simulink model "Traffic_Light"  (R2022b)
settings: Solver=VariableStepAuto  StartTime=0.0  StopTime=50  RelTol=1e-3
settings Model: Creator=MAAM  LastModifiedBy=MAAM

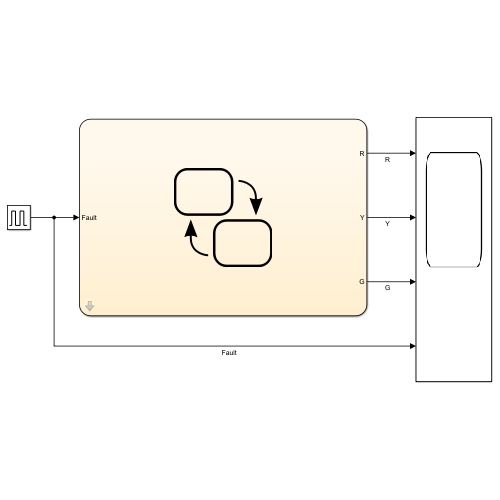
[thumbnail: Simulink's stored preview of the top-level diagram]
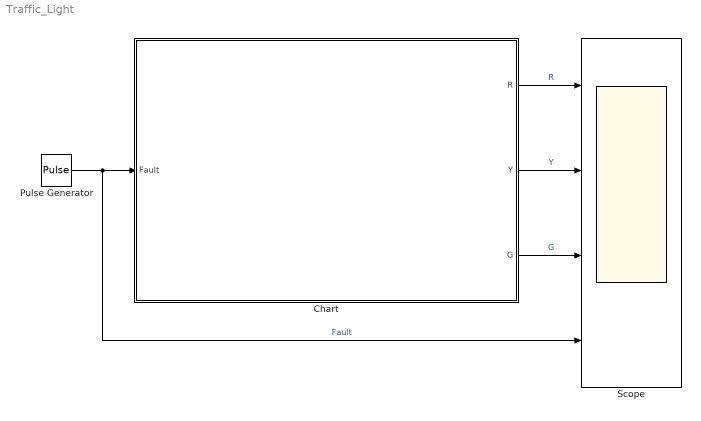
== system Traffic_Light ==
  Chart : Stateflow chart  TreatAsAtomicUnit=on  mask{GoTime=10, PrepTime=5, StopTime=2, ToggleTime=0.5}
  Pulse Generator : DiscretePulseGenerator  PulseType=Time based  Period=50  PulseWidth=30
  Scope : Scope  NumInputPorts=4
  wires:
  Chart/3(G) -> Scope/3  "G"
  Chart/1(R) -> Scope/1  "R"
  Chart/2(Y) -> Scope/2  "Y"
  Pulse Generator/1 -> Scope/4, Chart/1(Fault)  "Fault"

== stateflow chart Traffic_Light/Chart ==
  state Normal
    state Go
      en:
      G=true;
      ex:
      G=false;
    state PrepareToStop
      en:
      Y=true;
      ex:
      Y=false;
    state Stop
      en:
      R=true;
      ex:
      R=false;
    (default) -> Stop
    PrepareToStop -> Stop : after(PrepTime, sec)
    Go -> PrepareToStop : after(GoTime, sec)
    Stop -> Go : after(StopTime, sec)
  state Fault
    state Led_Off
      en:
      R=false;
      Y=false;
      G=false;
    state Led_On
      en:
      R=true;
      ex:
      R=false;
    (default) -> Led_Off
    Led_Off -> Led_On : after(ToggleTime, sec)
    Led_On -> Led_Off : after(ToggleTime, sec)
  (default) -> Normal
  Normal -> Fault : [Fault]
  Fault -> Normal : [Fault ~= true]
  data: Fault input; GoTime parameter; PrepTime parameter; StopTime parameter; R output; Y output; G output; ToggleTime parameter
